simulink model "regulatorsim"  (Simulink 5.0)
settings: Solver=ode45  StartTime=0.0  StopTime=Tstop  RelTol=1e-3
values from neighbouring files (symbols this model uses):
  Cimp = lincon(model,'reg',weights,interval,limits)    [doubleint.m]    (also in doubleintexp.m; example2.m = lincon(model,'track',cost,interval,limits); mexexample1.m = lincon(sysd,'track',cost,interval,limits); regsiso.m)
  x10 = 2    [regulator.m]
  x20 = 3    [regulator.m]
libraries: hyblib x1, simulink x1
settings Model: LastModifiedBy=Xbemporad

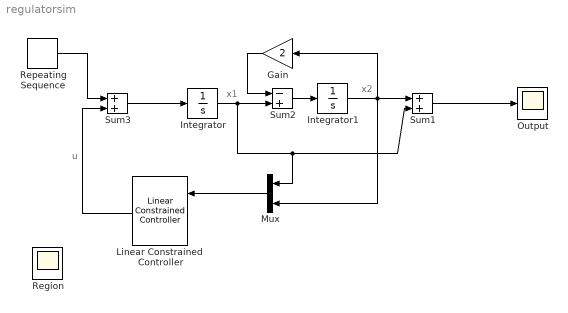
== system regulatorsim ==
  note: x2
  note: x1
  note: u
  Gain : Gain  Orientation=left  Gain=2  SaturateOnIntegerOverflow=on
  Integrator : Integrator  InitialCondition=x10
  Integrator1 : Integrator  InitialCondition=x20
  Linear Constrained  Controller : hyblib/Linear Constrained  Controller  Orientation=left  AncestorBlock=|  C=Cimp  xhat0=[]  u1=[]
      | hyblib/Controller for Constrained
      | Linear Systems (y,r)
  Mux : Mux  Orientation=left  Inputs=2
  Output : Scope
      settings: TimeRange=30  YMax=10
  Region : Scope
  Repeating Sequence : simulink/Sources/Repeating Sequence  rep_seq_t=[0 .1 10]  rep_seq_y=[100 0 0]
  Sum1 : Sum  SaturateOnIntegerOverflow=on
  Sum2 : Sum  Inputs=-+  SaturateOnIntegerOverflow=on
  Sum3 : Sum  SaturateOnIntegerOverflow=on
  wires:
  Mux/1 -> Linear Constrained  Controller/1
  Integrator1/1 -> Gain/1, Sum1/1, Mux/2
  Sum2/1 -> Integrator1/1
  Integrator/1 -> Sum2/2, Sum1/2, Mux/1
  Gain/1 -> Sum2/1
  Sum1/1 -> Output/1
  Repeating Sequence/1 -> Sum3/1
  Sum3/1 -> Integrator/1
  Linear Constrained  Controller/1 -> Sum3/2
